simulink model "test_2018"  (R2021b)
settings: Solver=VariableStepAuto  StartTime=0.0  StopTime=25  RelTol=1e-3
PreLoadFcn:
  | load("table_calibration.mat")
undefined symbols (not defined in the file or in its folder): aubr, tablebr, vubr
libraries: Solver_SF x1
settings Model: Creator=Lenovo  LastModifiedBy=sk
settings SolverCC: AlgebraicLoopSolver=TrustRegion
settings DebuggingCC: UnconnectedInputMsg=none  UnconnectedOutputMsg=none  UnconnectedLineMsg=none  SFMachineParentedDataDiag=warning  ArithmeticOperatorsInVariantConditions=warning
settings SFSimCC: CustomCodeUndefinedFunction=UseInterfaceOnly

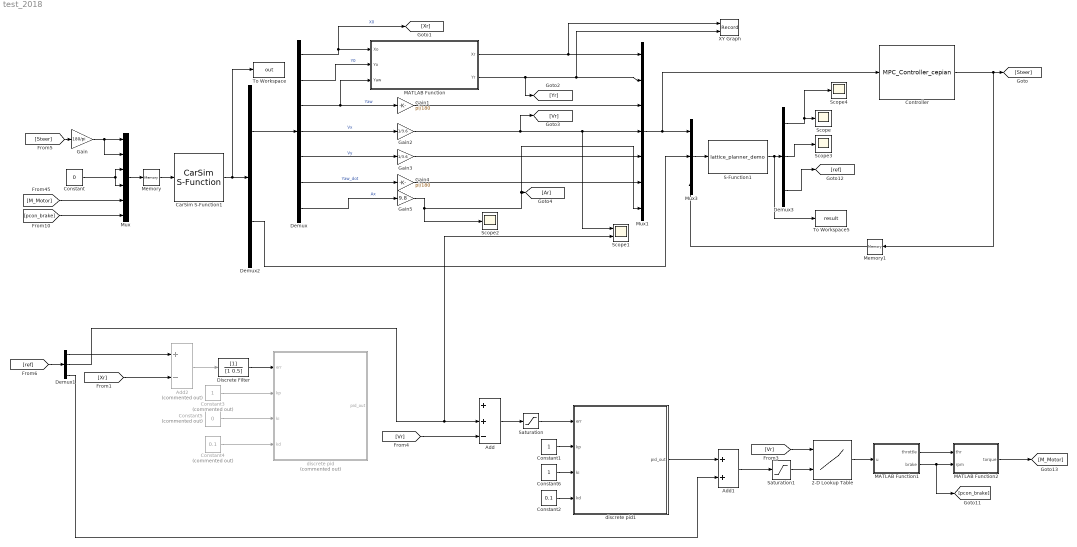
== system test_2018 ==
  2-D Lookup Table : Lookup_n-D  BreakpointsForDimension1=vubr  BreakpointsForDimension2=aubr  Table=tablebr  InternalRulePriority=Speed  RndMeth=Simplest  InputSameDT=on
      settings: InputPortMap=u0,u1
  Add : Sum  Inputs=++-
  Add1 : Sum
  Add2 : Sum  Commented=on  Inputs=+-
  CarSim S-Function1 : Solver_SF/CarSim S-Function  Priority=1  SIMFILE=simfile.sim  Run_RTs=off  vs_state_ind=Run  StopMode_ind=Vehicle Model
  Constant : Constant  Value=0
  Constant1 : Constant
  Constant2 : Constant  Value=0.1
  Constant3 : Constant  Commented=on
  Constant4 : Constant  Commented=on  Value=0.1
  Constant5 : Constant  Commented=on  Value=0
  Constant6 : Constant
  Controller : S-Function  FunctionName=MPC_Controller_cepian  SFunctionDeploymentMode=off  EnableBusSupport=off
  Demux : Demux  Outputs=7
  Demux1 : Demux  Outputs=3
  Demux2 : Demux  Outputs=[7 38]
  Demux3 : Demux  Outputs=[1 1 3]
  Discrete Filter : DiscreteFilter
  Gain : Gain  Gain=180/pi
  Gain1 : Gain  Gain=pi/180
  Gain2 : Gain  Gain=1/3.6
  Gain3 : Gain  Gain=1/3.6
  Gain4 : Gain  Gain=pi/180
  Gain5 : Gain  Gain=9.8
  MATLAB Function : MATLAB Function  TreatAsAtomicUnit=on
  MATLAB Function1 : MATLAB Function  TreatAsAtomicUnit=on
  MATLAB Function2 : MATLAB Function  TreatAsAtomicUnit=on
  Memory : Memory
  Memory1 : Memory
  Mux : Mux  Inputs=6
  Mux1 : Mux  Inputs=7
  Mux3 : Mux  Inputs=3
  S-Function1 : S-Function  FunctionName=lattice_planner_demo  SFunctionDeploymentMode=off  EnableBusSupport=off
  Saturation : Saturate  UpperLimit=45  LowerLimit=-45
  Saturation1 : Saturate  UpperLimit=5  LowerLimit=-8
  Scope{,2..4} (4 alike) : Scope
  Scope1 : Scope  NumInputPorts=2
  To Workspace : ToWorkspace  VariableName=out  SaveFormat=Structure With Time  SampleTime=-1
  To Workspace5 : ToWorkspace  VariableName=result  SaveFormat=Timeseries  SampleTime=-1
  XY Graph : Record  FileSettingsInternal="{\"entries\":[{\"content\":{\"excelSettings\":{\"content\":{},\"type\":\"Streamout.ExcelSettings\"}},\"type\":\"Streamout.FileSettingStorage\",\"uuid\":\"055e184a-daf4-4550-9570-af5b8ba2bb29\"}],\"packageUris\":[\"http://schema.mathworks.com/mf0/streamout_blocks/R2020a\"],\"version\":\"1.0\"}"  Layout=[1 1]  SignalsInternal="{\"entries\":[{\"content\":{\"signals\":[{\"content\":{\"blockPath\":[\"test_2018/XY Graph\"],\"channel\":[],\"dimensions\":[1],\"domain\":\"test_2018/XY Graph\",\"lineColor\":\"#a2142f\",\"plots\":[1],\"port\":1,\"sid\":[\"\"],\"signalID\":87719,\"signalName\":\"MATLAB Function:1\"},\"type\":\"RecordBlkView.Signal\",\"uuid\":\"ef74e0c8-c76b-4fb3-8589-69f741852af8\"},{\"content\":{\"blockPath\":[\"test_2018/XY Graph\"],\"channel\":[],\"dimensions\":[1],\"domain\":\"test_2018/XY Graph\",\"lineColor\":\"#139fff\",\"plots\":[1],\"port\":2,\"sid\":[\"\"],\"signalID\":87723,\"signalName\":\"MATLAB Function:2\"},\"type\":\"RecordBlkView.Signal\",\"uuid\":\"9884fad7-1a8f-43e4-be29-c34825d1d259\"}]},\"type\":\"RecordBlkView.InputSignals\",\"uuid\":\"8637a28f-95fb-4425-9f36-c1fa59b6d7f3\"}],\"packageUris\":[\"http://schema.mathworks.com/mf0/streamout_blocks/R2020a\"],\"version\":\"1.0\"}"  VisualizationBindings="{\"xyplotplugin\":{\"info\":[{\"series\":[{\"bindingParametersList\":[{\"parameter\":\"X-Axis\",\"signalID\":87719,\"signalName\":\"MATLAB Function:1\"},{\"parameter\":\"Y-Axis\",\"signalID\":87723,\"signalName\":\"MATLAB Function:2\"}],\"seriesID\":57691}],\"subplotID\":1}]}}"  CompatibilityTag=XY  st=-1
  discrete pid : Subsystem  Commented=on
  discrete pid1 : Subsystem
  wires:
  Mux/1 -> Memory/1
  Demux/3 -> Gain1/1, MATLAB Function/3(Yaw)  "Yaw"
  Demux/6 -> Gain4/1  "Yaw_dot"
  Demux/5 -> Gain3/1  "Vy"
  Demux/4 -> Gain2/1  "Vx"
  Demux/1 -> [Xr], MATLAB Function/1(Xo)  "X0"
  Gain1/1 -> Mux1/3
  Gain3/1 -> Mux1/5
  Gain4/1 -> Mux1/6
  Controller/1 -> Memory1/1, [Steer]
  Demux/7 -> Gain5/1  "Ax"
  Gain5/1 -> Scope2/1, [Ar], Mux1/7
  Mux1/1 -> Controller/1, Mux3/1
  S-Function1/1 -> To Workspace5/1, Demux3/1
  Memory/1 -> CarSim S-Function1/1
  Demux2/1 -> Demux/1
  Demux2/2 -> Mux3/2
  Mux3/1 -> S-Function1/1
  Memory1/1 -> Mux3/3
  Demux1/3 -> Add1/2
  Constant1/1 -> discrete pid1/2(kp)
  Constant2/1 -> discrete pid1/4(kd)
  Add/1 -> Saturation/1
  Constant4/1 -> discrete pid/4(kd)
  Constant6/1 -> discrete pid1/3(ki)
  Constant5/1 -> discrete pid/3(ki)
  Saturation1/1 -> 2-D Lookup Table/2
  Add2/1 -> Discrete Filter/1
  Add1/1 -> Saturation1/1
  Constant3/1 -> discrete pid/2(kp)
  2-D Lookup Table/1 -> MATLAB Function1/1(u)
  discrete pid1/1(pid_out) -> Add1/1
  Demux1/2 -> Scope1/2, Add/2
  Saturation/1 -> discrete pid1/1(err)
  Demux1/1 -> Add2/1
  Gain2/1 -> [Vr], Scope1/1, Mux1/4
  MATLAB Function1/1(throttle) -> MATLAB Function2/1(thr)
  MATLAB Function1/2(brake) -> [pcon_brake], MATLAB Function2/2(rpm)
  MATLAB Function/2(Yr) -> [Yr], Mux1/2, XY Graph/2
  MATLAB Function/1(Xr) -> XY Graph/1, Mux1/1
  Demux/2 -> MATLAB Function/2(Yo)  "Y0"
  [M_Motor] -> Mux/5
  [pcon_brake] -> Mux/6
  MATLAB Function2/1(torque) -> [M_Motor]
  [Steer] -> Gain/1
  [Vr] -> 2-D Lookup Table/1
  [Xr] -> Add2/2
  Discrete Filter/1 -> discrete pid/1(err)
  Constant/1 -> Mux/4, Mux/3
  [ref] -> Demux1/1
  [Vr] -> Add/3
  Gain/1 -> Mux/2, Mux/1
  Demux3/1 -> Scope4/1, Scope/1
  Demux3/2 -> Scope3/1
  Demux3/3 -> [ref]
  CarSim S-Function1/1 -> To Workspace/1, Demux2/1

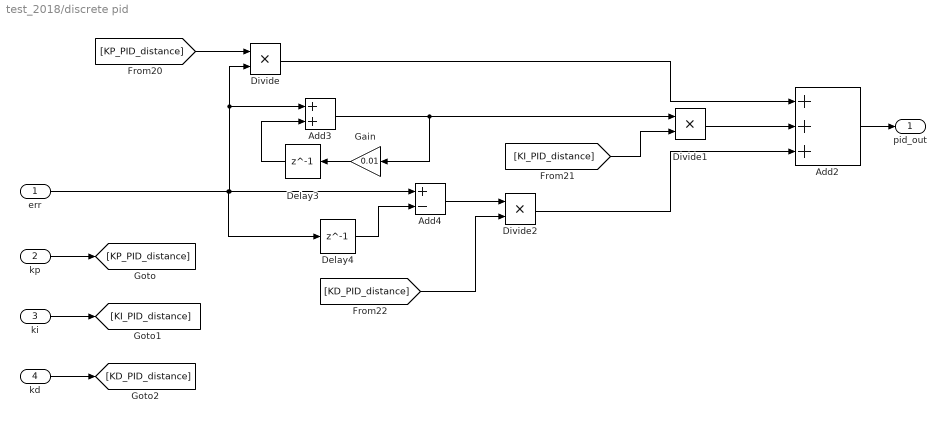
== system test_2018/discrete pid ==
  err : Inport
  kp : Inport  Port=2
  ki : Inport  Port=3
  kd : Inport  Port=4
  Add2 : Sum  Inputs=+++
  Add3 : Sum
  Add4 : Sum  Inputs=+-
  Delay3 : Delay  DelayLength=1
  Delay4 : Delay  DelayLength=1
  Divide : Product  Inputs=**
  Divide1 : Product  Inputs=**
  Divide2 : Product  Inputs=**
  Gain : Gain  Gain=0.01
  pid_out : Outport
  wires:
  [KD_PID_distance] -> Divide2/2
  err/1 -> Delay4/1, Divide/2, Add3/1, Add4/1
  Divide/1 -> Add2/1
  Divide2/1 -> Add2/3
  Add3/1 -> Gain/1, Divide1/1
  Delay4/1 -> Add4/2
  [KP_PID_distance] -> Divide/1
  Divide1/1 -> Add2/2
  Delay3/1 -> Add3/2
  [KI_PID_distance] -> Divide1/2
  Add4/1 -> Divide2/1
  Add2/1 -> pid_out/1
  kp/1 -> [KP_PID_distance]
  ki/1 -> [KI_PID_distance]
  kd/1 -> [KD_PID_distance]
  Gain/1 -> Delay3/1

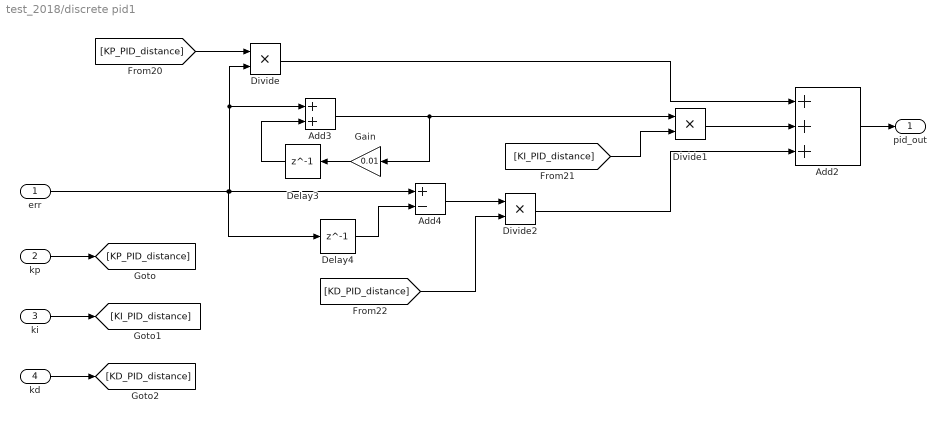
== system test_2018/discrete pid1 ==
  err : Inport
  kp : Inport  Port=2
  ki : Inport  Port=3
  kd : Inport  Port=4
  Add2 : Sum  Inputs=+++
  Add3 : Sum
  Add4 : Sum  Inputs=+-
  Delay3 : Delay  DelayLength=1
  Delay4 : Delay  DelayLength=1
  Divide : Product  Inputs=**
  Divide1 : Product  Inputs=**
  Divide2 : Product  Inputs=**
  Gain : Gain  Gain=0.01
  pid_out : Outport
  wires:
  Gain/1 -> Delay3/1
  kd/1 -> [KD_PID_distance]
  ki/1 -> [KI_PID_distance]
  kp/1 -> [KP_PID_distance]
  Add2/1 -> pid_out/1
  Add4/1 -> Divide2/1
  [KI_PID_distance] -> Divide1/2
  Delay3/1 -> Add3/2
  Divide1/1 -> Add2/2
  [KP_PID_distance] -> Divide/1
  Delay4/1 -> Add4/2
  Add3/1 -> Divide1/1, Gain/1
  Divide2/1 -> Add2/3
  Divide/1 -> Add2/1
  err/1 -> Add4/1, Add3/1, Divide/2, Delay4/1
  [KD_PID_distance] -> Divide2/2

== matlab function test_2018/MATLAB Function2 ==
  data: thr input; torque output; rpm input
function torque = fcn(thr,rpm)
Tmax=380*thr;
    if (rpm<=4523)
        torque=Tmax;
    else
        torque=Tmax*4523/rpm;
    end
end

== matlab function test_2018/MATLAB Function ==
  data: Xo input; Xr output; Yo input; Yaw input; Yr output
function [Xr,Yr] = fcn(Xo,Yo,Yaw)
l=2.77622;%轴距
Xr=Xo-l*cos(Yaw/180*pi);
Yr=Yo-l*sin(Yaw/180*pi);

== matlab function test_2018/MATLAB Function1 ==
  data: u input; throttle output; brake output
function [throttle,brake] = fcn(u)
    if u>=0
        throttle=u;
        brake=0;
    else
        throttle=0;
        brake=-u;
    end
